simulink model "BLDC_Motor_Plant"  (R2020b)
settings: Solver=VariableStepAuto  StartTime=0.0  StopTime=10.0  RelTol=1e-3
model workspace (MAT data in the model file):
  den = [0.0001 0.014]
  den1 = [0.0002 0.004586]
  kT = 0.0275
  ke = 0.0275
  num = 1
  num1 = 1
settings Model: Creator=intel  LastModifiedBy=intel
settings DataIOCC: SaveOutput=off  SaveTime=off
settings DebuggingCC: AlgebraicLoopMsg=none

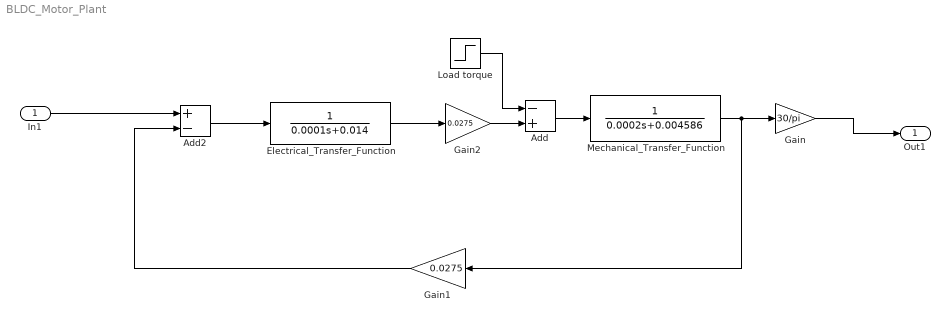
== system BLDC_Motor_Plant ==
  In1 : Inport  OutDataTypeStr=double  PortDimensions=1  SampleTime=0
  Add : Sum  Inputs=-+
  Add2 : Sum  Inputs=+-
  Electrical_Transfer_Function : TransferFcn  Denominator=[0.0001 0.014]
  Gain : Gain  Gain=30/pi
  Gain1 : Gain  Gain=0.0275
  Gain2 : Gain  Gain=0.0275
  Load torque : Step  SampleTime=0
  Mechanical_Transfer_Function : TransferFcn  Denominator=[0.0002 0.004586]
  Out1 : Outport  OutDataTypeStr=double  PortDimensions=1  SampleTime=0
  wires:
  Mechanical_Transfer_Function/1 -> Gain/1, Gain1/1
  Gain1/1 -> Add2/2
  Load torque/1 -> Add/1
  Add2/1 -> Electrical_Transfer_Function/1
  Gain2/1 -> Add/2
  Gain/1 -> Out1/1
  Add/1 -> Mechanical_Transfer_Function/1
  In1/1 -> Add2/1
  Electrical_Transfer_Function/1 -> Gain2/1
